simulink model "THD_multilevel_singlephase"  (R2015a)
settings: Solver=ode45  StartTime=0.02  StopTime=0.04  RelTol=1e-3
libraries: simulink x27, powerlib_meascontrol x24, powerlib x21
settings Model: Creator=Yahya  LastModifiedBy=Yahya

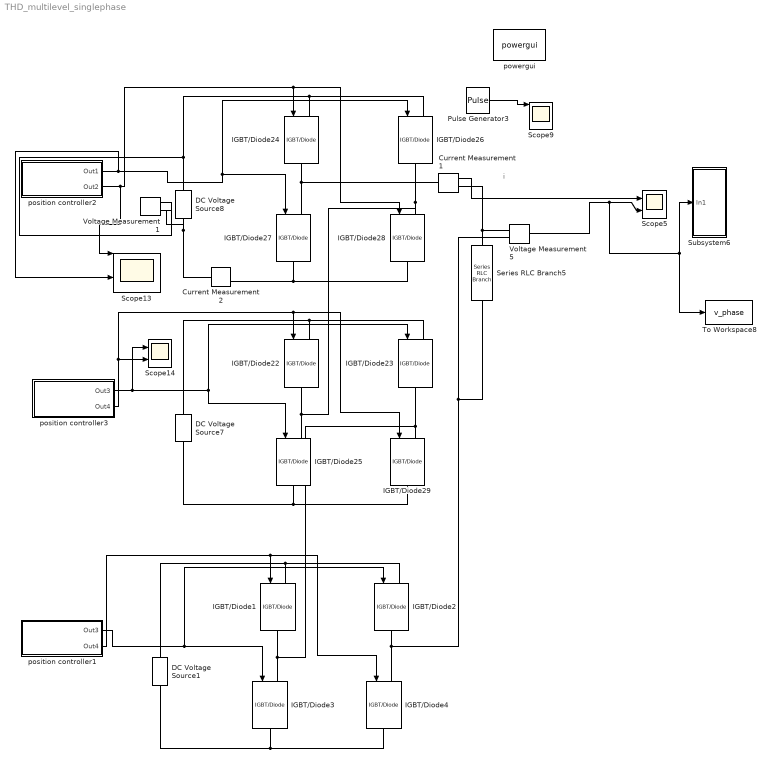
== system THD_multilevel_singlephase ==
  note: i
  Current Measurement1 : powerlib/Measurements/Current Measurement  PhasorSimulation=off  OutputType=Complex  PSBequivalent=0
  Current Measurement2 : powerlib/Measurements/Current Measurement  PhasorSimulation=off  OutputType=Complex  PSBequivalent=0
  DC Voltage Source1 : powerlib/Electrical Sources/DC Voltage Source  Amplitude=100  Measurements=None
  DC Voltage Source7 : powerlib/Electrical Sources/DC Voltage Source  Amplitude=100  Measurements=None
  DC Voltage Source8 : powerlib/Electrical Sources/DC Voltage Source  Amplitude=100  Measurements=None
  IGBT/Diode{1..4,22..29} (12 alike) : powerlib/Power Electronics/IGBT//Diode  Ron=1e-3  Rs=1e5  Cs=inf  Measurements=off
  Pulse Generator3 : DiscretePulseGenerator  PulseType=Time based  Amplitude=0.8  Period=0.00001  PulseWidth=50
  Scope13 : Scope  NumInputPorts=6
      settings: TimeRange=0.2  YMin=190~-5~-5~-5~-5~-5  YMax=400~5~5~5~5~5  SaveName=ScopeData25
  Scope14 : Scope  NumInputPorts=2
      settings: TimeRange=0.2  YMin=190~-5  YMax=400~5  SaveName=ScopeData26
  Scope5 : Scope  NumInputPorts=2
      settings: TimeRange=1  YMin=-400~-400  YMax=400~400  SaveName=ScopeData3
  Scope9 : Scope  NumInputPorts=4
      settings: YMin=-5~-5~-5~-5  YMax=5~5~5~5  SaveName=ScopeData18
  Series RLC Branch5 : powerlib/Elements/Series RLC Branch  LConnTagsString=__new0  RConnTagsString=__new0  BranchType=RL  Resistance=1.405*2  Inductance=0.005839*2  SetiL0=off  InitialCurrent=0  Capacitance=1e-6  Setx0=off  InitialVoltage=0  Measurements=None
  Subsystem6 : Subsystem
  To Workspace8 : ToWorkspace  VariableName=v_phase  SaveFormat=Timeseries  SampleTime=-1
  Voltage Measurement1 : powerlib/Measurements/Voltage Measurement  PhasorSimulation=off  OutputType=Complex  PSBequivalent=0
  Voltage Measurement5 : powerlib/Measurements/Voltage Measurement  PhasorSimulation=off  OutputType=Complex  PSBequivalent=0
  position controller1 : Subsystem
  position controller2 : Subsystem
  position controller3 : Subsystem
  powergui : powerlib/powergui  Priority=1  SimulationMode=Continuous  SolverType=Tustin/Backward Euler (TBE)  SampleTime=50e-6  frequency=60  SPID=off  DisableSnubberDevices=off  DisableRonSwitches=off  DisableVfSwitches=off  SwTol=0  DisplayEquations=off  Interpol=off  methode=off  Ts=100  FunctionMessages=off  echomessages=off  HookPort=off  EnableUseOfTLC=off  x0status=blocks  frequencyindice=0  Pbase=100e6  ErrMax=1e-4  Iterations=50  UnitsV=kV  UnitsW=MW  buscounter=0  RestoreLinks=warning  ResistiveCurrentMeasurement=off  Frange=[0:2:500]  Ylog=off  Xlog=on  ShowGrid=off  save=off  variable=ZData  structure=0  ZoomFFT=off  StartTime=0.0  cycles=1  DisplayStyle=1  fundamental=60  FreqAxis=off  MaxFrequency=1000  frequencyindicesteady=1  RmsSteady=1  display=off
  wires:
  position controller2/2(Out2) -> Scope13/1, IGBT/Diode28/1, IGBT/Diode24/1
  position controller2/1(Out1) -> Scope13/4, IGBT/Diode26/1, IGBT/Diode27/1
  position controller3/2(Out4) -> Scope14/2, IGBT/Diode29/1, IGBT/Diode22/1
  Current Measurement1/1 -> Scope5/1
  position controller1/2(Out4) -> IGBT/Diode4/1, IGBT/Diode1/1
  position controller1/1(Out3) -> IGBT/Diode3/1, IGBT/Diode2/1
  Voltage Measurement5/1 -> To Workspace8/1, Subsystem6/1(In1), Scope5/2
  Pulse Generator3/1 -> Scope9/1
  position controller3/1(Out3) -> Scope14/1, IGBT/Diode23/1, IGBT/Diode25/1
  connections:
  IGBT/Diode24/LConn1 -- DC Voltage Source8/RConn1 -- Voltage Measurement1/LConn2 -- IGBT/Diode26/LConn1
  IGBT/Diode27/RConn1 -- IGBT/Diode28/RConn1 -- Current Measurement2/RConn1
  Current Measurement1/LConn1 -- IGBT/Diode24/RConn1 -- IGBT/Diode27/LConn1
  IGBT/Diode22/LConn1 -- DC Voltage Source7/RConn1 -- IGBT/Diode23/LConn1
  IGBT/Diode25/RConn1 -- DC Voltage Source7/LConn1 -- IGBT/Diode29/RConn1
  IGBT/Diode26/RConn1 -- IGBT/Diode28/LConn1 -- IGBT/Diode22/RConn1 -- IGBT/Diode25/LConn1
  IGBT/Diode1/RConn1 -- IGBT/Diode3/LConn1 -- IGBT/Diode29/LConn1 -- IGBT/Diode23/RConn1
  Current Measurement1/RConn1 -- Voltage Measurement5/LConn1 -- Series RLC Branch5/LConn1
  IGBT/Diode2/LConn1 -- IGBT/Diode1/LConn1 -- DC Voltage Source1/RConn1
  IGBT/Diode4/RConn1 -- IGBT/Diode3/RConn1 -- DC Voltage Source1/LConn1
  Series RLC Branch5/RConn1 -- IGBT/Diode4/LConn1 -- IGBT/Diode2/RConn1 -- Voltage Measurement5/LConn2
  Voltage Measurement1/LConn1 -- DC Voltage Source8/LConn1 -- Current Measurement2/LConn1

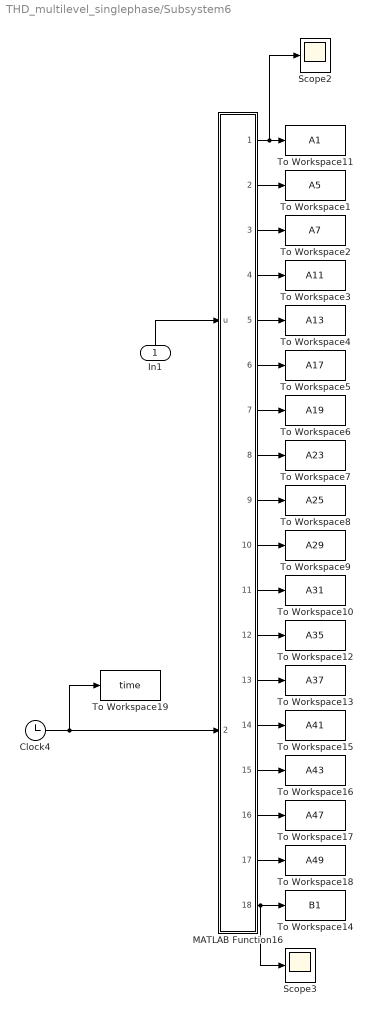
== system THD_multilevel_singlephase/Subsystem6 ==
  In1 : Inport
  Clock4 : Clock
  MATLAB Function16 : MATLAB Function  TreatAsAtomicUnit=on
  Scope2 : Scope
      settings: TimeRange=0.2  YMin=190  YMax=400  SaveName=ScopeData7
  Scope3 : Scope
      settings: TimeRange=0.2  YMin=190  YMax=400  SaveName=ScopeData9
  To Workspace1 : ToWorkspace  VariableName=A5  SaveFormat=Timeseries  SampleTime=-1
  To Workspace10 : ToWorkspace  VariableName=A31  SaveFormat=Timeseries  SampleTime=-1
  To Workspace11 : ToWorkspace  VariableName=A1  SaveFormat=Timeseries  SampleTime=-1
  To Workspace12 : ToWorkspace  VariableName=A35  SaveFormat=Timeseries  SampleTime=-1
  To Workspace13 : ToWorkspace  VariableName=A37  SaveFormat=Timeseries  SampleTime=-1
  To Workspace14 : ToWorkspace  VariableName=B1  SaveFormat=Timeseries  SampleTime=-1
  To Workspace15 : ToWorkspace  VariableName=A41  SaveFormat=Timeseries  SampleTime=-1
  To Workspace16 : ToWorkspace  VariableName=A43  SaveFormat=Timeseries  SampleTime=-1
  To Workspace17 : ToWorkspace  VariableName=A47  SaveFormat=Timeseries  SampleTime=-1
  To Workspace18 : ToWorkspace  VariableName=A49  SaveFormat=Timeseries  SampleTime=-1
  To Workspace19 : ToWorkspace  VariableName=time  SaveFormat=Timeseries  SampleTime=-1
  To Workspace2 : ToWorkspace  VariableName=A7  SaveFormat=Timeseries  SampleTime=-1
  To Workspace3 : ToWorkspace  VariableName=A11  SaveFormat=Timeseries  SampleTime=-1
  To Workspace4 : ToWorkspace  VariableName=A13  SaveFormat=Timeseries  SampleTime=-1
  To Workspace5 : ToWorkspace  VariableName=A17  SaveFormat=Timeseries  SampleTime=-1
  To Workspace6 : ToWorkspace  VariableName=A19  SaveFormat=Timeseries  SampleTime=-1
  To Workspace7 : ToWorkspace  VariableName=A23  SaveFormat=Timeseries  SampleTime=-1
  To Workspace8 : ToWorkspace  VariableName=A25  SaveFormat=Timeseries  SampleTime=-1
  To Workspace9 : ToWorkspace  VariableName=A29  SaveFormat=Timeseries  SampleTime=-1
  wires:
  MATLAB Function16/1(A1) -> Scope2/1, To Workspace11/1
  Clock4/1 -> To Workspace19/1, MATLAB Function16/2(time)
  MATLAB Function16/4(A11) -> To Workspace3/1
  MATLAB Function16/2(A5) -> To Workspace1/1
  In1/1 -> MATLAB Function16/1(u)
  MATLAB Function16/3(A7) -> To Workspace2/1
  MATLAB Function16/5(A13) -> To Workspace4/1
  MATLAB Function16/6(A17) -> To Workspace5/1
  MATLAB Function16/7(A19) -> To Workspace6/1
  MATLAB Function16/8(A23) -> To Workspace7/1
  MATLAB Function16/9(A25) -> To Workspace8/1
  MATLAB Function16/10(A29) -> To Workspace9/1
  MATLAB Function16/11(A31) -> To Workspace10/1
  MATLAB Function16/12(A35) -> To Workspace12/1
  MATLAB Function16/13(A37) -> To Workspace13/1
  MATLAB Function16/14(A41) -> To Workspace15/1
  MATLAB Function16/15(A43) -> To Workspace16/1
  MATLAB Function16/16(A47) -> To Workspace17/1
  MATLAB Function16/17(A49) -> To Workspace18/1
  MATLAB Function16/18(B1) -> To Workspace14/1, Scope3/1

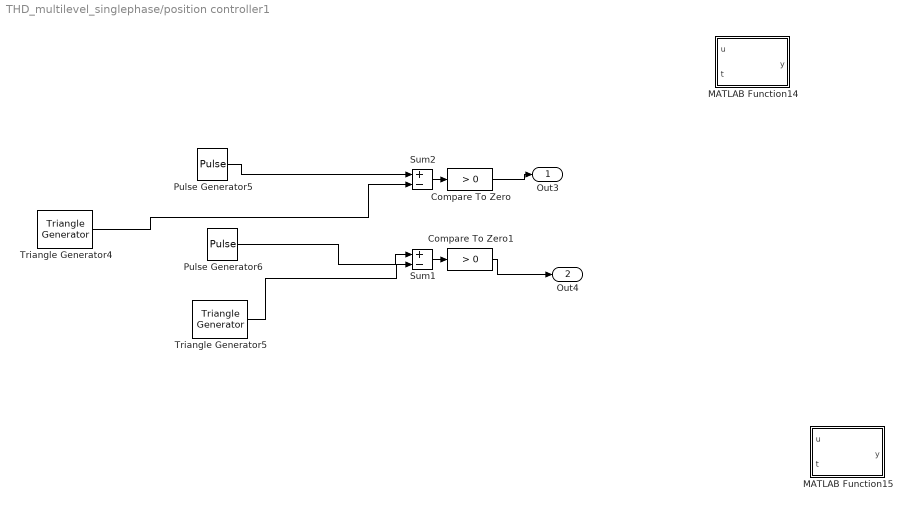
== system THD_multilevel_singlephase/position controller1 ==
  Compare To Zero : simulink/Logic and Bit Operations/Compare To Zero  relop=>  OutDataTypeStr=boolean  ZeroCross=off
  Compare To Zero1 : simulink/Logic and Bit Operations/Compare To Zero  relop=>  OutDataTypeStr=boolean  ZeroCross=off
  MATLAB Function14 : MATLAB Function  TreatAsAtomicUnit=on
  MATLAB Function15 : MATLAB Function  TreatAsAtomicUnit=on
  Pulse Generator5 : DiscretePulseGenerator  PulseType=Time based  Amplitude=0.127819930463041  Period=0.02  PulseWidth=50.001
  Pulse Generator6 : DiscretePulseGenerator  PulseType=Time based  Amplitude=0.127819930463041  Period=0.02  PulseWidth=50.001  PhaseDelay=0.01
  Sum1 : Sum  Inputs=+-  OutDataTypeStr=double
  Sum2 : Sum  Inputs=+-  OutDataTypeStr=double
  Triangle Generator4 : powerlib_meascontrol/Pulse & Signal Generators/Triangle Generator  Freq=50  Phase=90  Ts=0
  Triangle Generator5 : powerlib_meascontrol/Pulse & Signal Generators/Triangle Generator  Freq=50  Phase=90+180  Ts=0
  Out3 : Outport
  Out4 : Outport  Port=2
  wires:
  Compare To Zero/1 -> Out3/1
  Compare To Zero1/1 -> Out4/1
  Triangle Generator4/1 -> Sum2/2
  Sum2/1 -> Compare To Zero/1
  Sum1/1 -> Compare To Zero1/1
  Pulse Generator5/1 -> Sum2/1
  Pulse Generator6/1 -> Sum1/1
  Triangle Generator5/1 -> Sum1/2

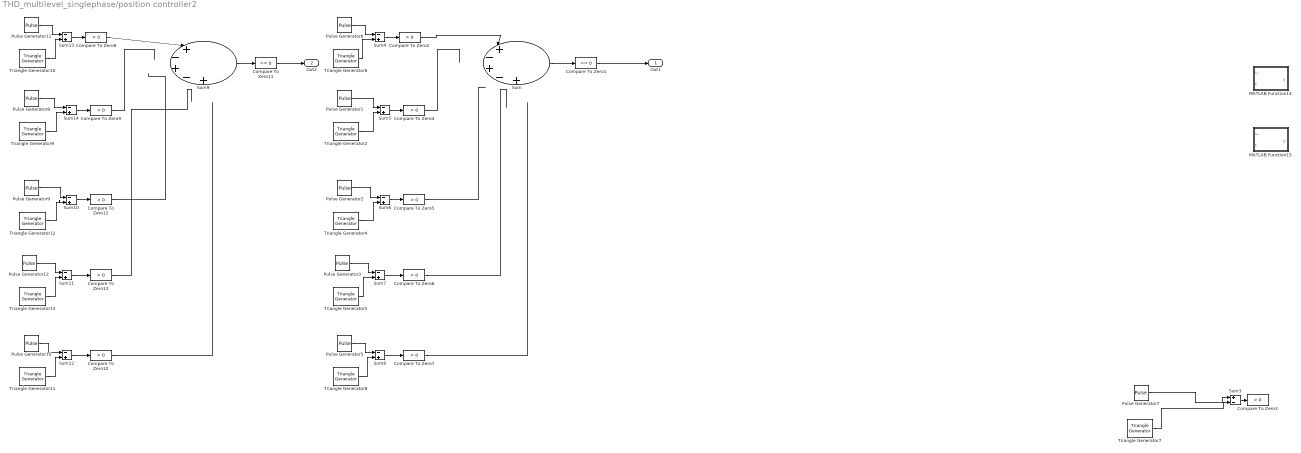
== system THD_multilevel_singlephase/position controller2 ==
  Compare To Zero1 : simulink/Logic and Bit Operations/Compare To Zero  relop===  OutDataTypeStr=boolean  ZeroCross=off
  Compare To Zero{2..10,12..13} (11 alike) : simulink/Logic and Bit Operations/Compare To Zero  relop=>  OutDataTypeStr=boolean  ZeroCross=off
  Compare To Zero11 : simulink/Logic and Bit Operations/Compare To Zero  relop===  OutDataTypeStr=boolean  ZeroCross=off
  MATLAB Function14 : MATLAB Function  TreatAsAtomicUnit=on
  MATLAB Function15 : MATLAB Function  TreatAsAtomicUnit=on
  Pulse Generator1 : DiscretePulseGenerator  PulseType=Time based  Amplitude=0.687674739965695  Period=0.02  PulseWidth=50.001
  Pulse Generator10 : DiscretePulseGenerator  PulseType=Time based  Amplitude=0.377812988041322  Period=0.02  PulseWidth=50.001  PhaseDelay=0.01
  Pulse Generator11 : DiscretePulseGenerator  PulseType=Time based  Amplitude=0.634629676981601  Period=0.02  PulseWidth=50.001  PhaseDelay=0.01
  Pulse Generator12 : DiscretePulseGenerator  PulseType=Time based  Amplitude=0.360085258924687  Period=0.02  PulseWidth=50.001  PhaseDelay=0.01
  Pulse Generator2 : DiscretePulseGenerator  PulseType=Time based  Amplitude=0.796099800558993  Period=0.02  PulseWidth=50.001
  Pulse Generator3 : DiscretePulseGenerator  PulseType=Time based  Amplitude=0.360085258924687  Period=0.02  PulseWidth=50.001
  Pulse Generator5 : DiscretePulseGenerator  PulseType=Time based  Amplitude=0.377812988041322  Period=0.02  PulseWidth=50.001
  Pulse Generator6 : DiscretePulseGenerator  PulseType=Time based  Amplitude=0.634629676981601  Period=0.02  PulseWidth=50.001
  Pulse Generator7 : DiscretePulseGenerator  PulseType=Time based  Amplitude=0.332  Period=0.02  PulseWidth=50  PhaseDelay=0.01
  Pulse Generator8 : DiscretePulseGenerator  PulseType=Time based  Amplitude=0.687674739965695  Period=0.02  PulseWidth=50.001  PhaseDelay=0.01
  Pulse Generator9 : DiscretePulseGenerator  PulseType=Time based  Amplitude=0.796099800558993  Period=0.02  PulseWidth=50.001  PhaseDelay=0.01
  Sum : Sum  Inputs=|+-+-+
  Sum{4..8,10..14} (10 alike) : Sum  Inputs=-+  OutDataTypeStr=double
  Sum3 : Sum  Inputs=+-  OutDataTypeStr=double
  Sum9 : Sum  Inputs=|+-+-+
  Triangle Generator{7,9..13} (6 alike) : powerlib_meascontrol/Pulse & Signal Generators/Triangle Generator  Freq=50  Phase=90+180  Ts=0
  Triangle Generator{2,4..6,8} (5 alike) : powerlib_meascontrol/Pulse & Signal Generators/Triangle Generator  Freq=50  Phase=90  Ts=0
  Out1 : Outport
  Out2 : Outport  Port=2
  wires:
  Triangle Generator6/1 -> Sum4/2
  Sum4/1 -> Compare To Zero2/1
  Sum3/1 -> Compare To Zero3/1
  Pulse Generator6/1 -> Sum4/1
  Pulse Generator7/1 -> Sum3/1
  Triangle Generator7/1 -> Sum3/2
  Triangle Generator2/1 -> Sum5/2
  Sum5/1 -> Compare To Zero4/1
  Pulse Generator1/1 -> Sum5/1
  Triangle Generator4/1 -> Sum6/2
  Sum6/1 -> Compare To Zero5/1
  Pulse Generator2/1 -> Sum6/1
  Triangle Generator5/1 -> Sum7/2
  Sum7/1 -> Compare To Zero6/1
  Pulse Generator3/1 -> Sum7/1
  Triangle Generator8/1 -> Sum8/2
  Sum8/1 -> Compare To Zero7/1
  Pulse Generator5/1 -> Sum8/1
  Compare To Zero2/1 -> Sum/1
  Compare To Zero5/1 -> ?
  Compare To Zero6/1 -> ?
  Compare To Zero7/1 -> ?
  Triangle Generator10/1 -> Sum13/2
  Sum13/1 -> Compare To Zero8/1
  Pulse Generator11/1 -> Sum13/1
  Triangle Generator9/1 -> Sum14/2
  Sum14/1 -> Compare To Zero9/1
  Pulse Generator8/1 -> Sum14/1
  Triangle Generator12/1 -> Sum10/2
  Sum10/1 -> Compare To Zero12/1
  Pulse Generator9/1 -> Sum10/1
  Triangle Generator13/1 -> Sum11/2
  Sum11/1 -> Compare To Zero13/1
  Pulse Generator12/1 -> Sum11/1
  Triangle Generator11/1 -> Sum12/2
  Sum12/1 -> Compare To Zero10/1
  Pulse Generator10/1 -> Sum12/1
  Compare To Zero8/1 -> Sum9/1
  Compare To Zero9/1 -> ?
  Compare To Zero12/1 -> ?
  Sum9/1 -> Compare To Zero11/1
  Compare To Zero13/1 -> ?
  Compare To Zero10/1 -> ?
  Compare To Zero4/1 -> ?
  Sum/1 -> Compare To Zero1/1
  Compare To Zero1/1 -> Out1/1
  Compare To Zero11/1 -> Out2/1

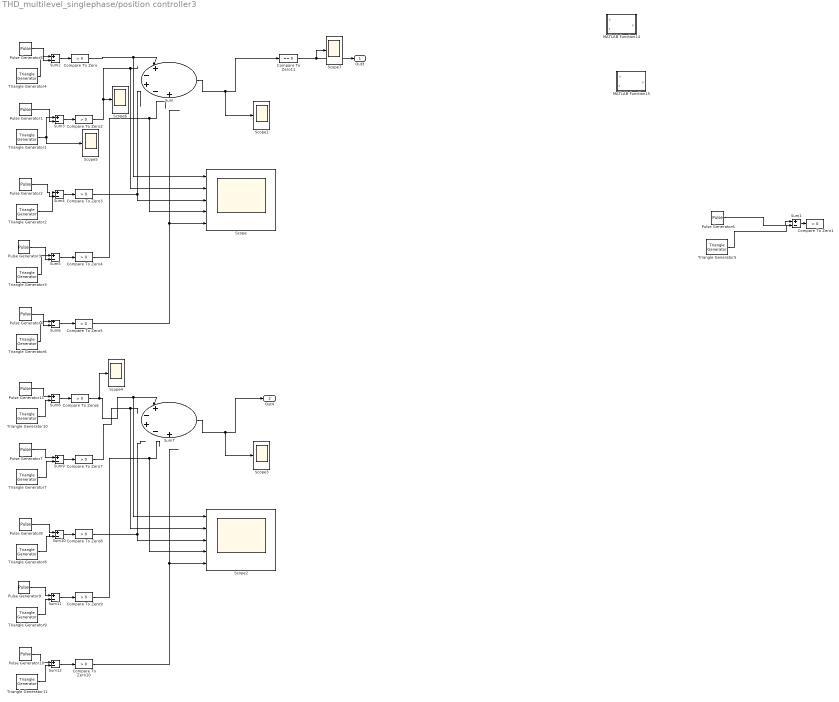
== system THD_multilevel_singlephase/position controller3 ==
  Compare To Zero{,1..10} (11 alike) : simulink/Logic and Bit Operations/Compare To Zero  relop=>  OutDataTypeStr=boolean  ZeroCross=off
  Compare To Zero11 : simulink/Logic and Bit Operations/Compare To Zero  relop===  OutDataTypeStr=boolean  ZeroCross=off
  MATLAB Function14 : MATLAB Function  TreatAsAtomicUnit=on
  MATLAB Function15 : MATLAB Function  TreatAsAtomicUnit=on
  Pulse Generator1 : DiscretePulseGenerator  PulseType=Time based  Amplitude=0.372911525752630  Period=0.02  PulseWidth=50.001
  Pulse Generator10 : DiscretePulseGenerator  PulseType=Time based  Amplitude=0.377812988041322  Period=0.02  PulseWidth=50.001  PhaseDelay=0.01
  Pulse Generator11 : DiscretePulseGenerator  PulseType=Time based  Amplitude=0.319276011251811  Period=0.02  PulseWidth=50.001  PhaseDelay=0.01
  Pulse Generator2 : DiscretePulseGenerator  PulseType=Time based  Amplitude=0.399283235379700  Period=0.02  PulseWidth=50.001
  Pulse Generator3 : DiscretePulseGenerator  PulseType=Time based  Amplitude=0.360085258924687  Period=0.02  PulseWidth=50.001
  Pulse Generator4 : DiscretePulseGenerator  PulseType=Time based  Amplitude=0.377812988041322  Period=0.02  PulseWidth=50.001
  Pulse Generator5 : DiscretePulseGenerator  PulseType=Time based  Amplitude=0.319276011251811  Period=0.02  PulseWidth=50.001
  Pulse Generator6 : DiscretePulseGenerator  PulseType=Time based  Amplitude=0.332  Period=0.02  PulseWidth=50  PhaseDelay=0.01
  Pulse Generator7 : DiscretePulseGenerator  PulseType=Time based  Amplitude=0.372911525752630  Period=0.02  PulseWidth=50.001  PhaseDelay=0.01
  Pulse Generator8 : DiscretePulseGenerator  PulseType=Time based  Amplitude=0.399283235379700  Period=0.02  PulseWidth=50.001  PhaseDelay=0.01
  Pulse Generator9 : DiscretePulseGenerator  PulseType=Time based  Amplitude=0.360085258924687  Period=0.02  PulseWidth=50.001  PhaseDelay=0.01
  Scope : Scope  NumInputPorts=5
      settings: TimeRange=0.02  YMin=0~0~0~0~0  YMax=1~1~1~1~1
  Scope{1,3..7} (6 alike) : Scope
      Scope1 settings: SaveName=ScopeData2
      Scope3 settings: SaveName=ScopeData5
      Scope4 settings: SaveName=ScopeData15
      Scope5 settings: SaveName=ScopeData6
      Scope6 settings: SaveName=ScopeData10
      Scope7 settings: SaveName=ScopeData11
  Scope2 : Scope  NumInputPorts=5
      settings: YMin=-5~-5~-5~-5~-5  YMax=5~5~5~5~5  SaveName=ScopeData4
  Sum : Sum  Inputs=|+-+-+
  Sum{1..6,8..12} (11 alike) : Sum  Inputs=+-  OutDataTypeStr=double
  Sum7 : Sum  Inputs=|+-+-+
  Triangle Generator{1..4,6} (5 alike) : powerlib_meascontrol/Pulse & Signal Generators/Triangle Generator  Freq=50  Phase=90  Ts=0
  Triangle Generator{5,7..11} (6 alike) : powerlib_meascontrol/Pulse & Signal Generators/Triangle Generator  Freq=50  Phase=90+180  Ts=0
  Out3 : Outport
  Out4 : Outport  Port=2
  wires:
  Triangle Generator4/1 -> Sum2/1
  Sum2/1 -> Compare To Zero/1
  Sum1/1 -> Compare To Zero1/1
  Pulse Generator5/1 -> Sum2/2
  Pulse Generator6/1 -> Sum1/1
  Triangle Generator5/1 -> Sum1/2
  Triangle Generator1/1 -> Sum3/1, Scope5/1
  Sum3/1 -> Compare To Zero2/1
  Pulse Generator1/1 -> Sum3/2
  Triangle Generator2/1 -> Sum4/1
  Sum4/1 -> Compare To Zero3/1
  Pulse Generator2/1 -> Sum4/2
  Triangle Generator3/1 -> Sum5/1
  Sum5/1 -> Compare To Zero4/1
  Pulse Generator3/1 -> Sum5/2
  Triangle Generator6/1 -> Sum6/1
  Sum6/1 -> Compare To Zero5/1
  Pulse Generator4/1 -> Sum6/2
  Compare To Zero/1 -> Scope/1, Sum/1
  Compare To Zero3/1 -> Scope/3
  Sum/1 -> Scope1/1, Compare To Zero11/1
  Compare To Zero4/1 -> Scope/4
  Compare To Zero5/1 -> Scope/5
  Triangle Generator10/1 -> Sum8/2
  Sum8/1 -> Compare To Zero6/1
  Pulse Generator11/1 -> Sum8/1
  Triangle Generator7/1 -> Sum9/2
  Sum9/1 -> Compare To Zero7/1
  Pulse Generator7/1 -> Sum9/1
  Triangle Generator8/1 -> Sum10/2
  Sum10/1 -> Compare To Zero8/1
  Pulse Generator8/1 -> Sum10/1
  Triangle Generator9/1 -> Sum11/2
  Sum11/1 -> Compare To Zero9/1
  Pulse Generator9/1 -> Sum11/1
  Triangle Generator11/1 -> Sum12/2
  Sum12/1 -> Compare To Zero10/1
  Pulse Generator10/1 -> Sum12/1
  Compare To Zero6/1 -> Scope4/1, Scope2/1, Sum7/1
  Compare To Zero7/1 -> Scope2/2
  Compare To Zero8/1 -> Scope2/3
  Sum7/1 -> Out4/1, Scope3/1
  Compare To Zero9/1 -> Scope2/4
  Compare To Zero10/1 -> Scope2/5
  Compare To Zero2/1 -> Scope/2, Scope6/1
  Compare To Zero11/1 -> Scope7/1, Out3/1

== matlab function THD_multilevel_singlephase/position controller3/MATLAB Function14 ==
  data: u input; y output; t input
function y = fcn(u,t)
%#codegen
if t>u
    y = 1;
else
    y = 0;
end
end

== matlab function THD_multilevel_singlephase/position controller2/MATLAB Function14 ==
  data: u input; y output; t input
function y = fcn(u,t)
%#codegen
if t>u
    y = 1;
else
    y = 0;
end
end

== matlab function THD_multilevel_singlephase/position controller1/MATLAB Function14 ==
  data: u input; y output; t input
function y = fcn(u,t)
%#codegen
if t>u
    y = 1;
else
    y = 0;
end
end

== matlab function THD_multilevel_singlephase/position controller2/MATLAB Function15 ==
  data: u input; y output; t input
function y = fcn(u,t)
%#codegen
if t>u
    y = 1;
else
    y = 0;
end
end

== matlab function THD_multilevel_singlephase/position controller1/MATLAB Function15 ==
  data: u input; y output; t input
function y = fcn(u,t)
%#codegen
if t>u
    y = 1;
else
    y = 0;
end
end

== matlab function THD_multilevel_singlephase/position controller3/MATLAB Function15 ==
  data: u input; y output; t input
function y = fcn(u,t)
%#codegen
if t>u
    y = 1;
else
    y = 0;
end
end

== matlab function THD_multilevel_singlephase/Subsystem6/MATLAB Function16 ==
  data: u input; A1 output; A5 output; A7 output; A11 output; A13 output; A17 output; A19 output; A23 output; A25 output; A29 output; A31 output; A35 output; A37 output; A41 output; A43 output; A47 output; A49 output; time input; B1 output
function [A1,A5,A7,A11,A13,A17,A19,A23,A25,A29,A31,A35,A37,A41,A43,A47,A49,B1] = fcn(u,time)
%#codegen
A1 = u*sin(2*pi*50*time);
A5 = u*sin(5*2*pi*50*time);
A7 = u*sin(7*2*pi*50*time);
A11 = u*sin(11*2*pi*50*time);
A13 = u*sin(13*2*pi*50*time);
A17 = u*sin(17*2*pi*50*time);
A19 = u*sin(19*2*pi*50*time);
A23 = u*sin(23*2*pi*50*time);
A25 = u*sin(25*2*pi*50*time);
A29 = u*sin(29*2*pi*50*time);
A31 = u*sin(31*2*pi*50*time);
A35 = u*sin(35*2*pi*50*time);
A37 = u*sin(37*2*pi*50*time);
A41 = u*sin(41*2*pi*50*time);
A43 = u*sin(43*2*pi*50*time);
A47 = u*sin(47*2*pi*50*time);
A49 = u*sin(49*2*pi*50*time);
B1 = u*cos(2*pi*50*time);
end
